simulink model "chap4_3sim"  (Simulink 6.3)
settings: Solver=ode45  StartTime=0.0  StopTime=10  FixedStep=0.001  RelTol=1e-3
libraries: simulink x1
settings Model: LastModifiedBy=Administrator  ExtModeTrigMode=oneshot  ExtModeArmWhenConnect=off  StrictBusMsg=None
settings DataIOCC: LimitDataPoints=off  SignalLoggingName=sigsOut
settings OptimizationCC: BooleanDataType=off
settings DebuggingCC: SolverPrmCheckMsg=none
settings HardwareCC: TargetUnknown=on

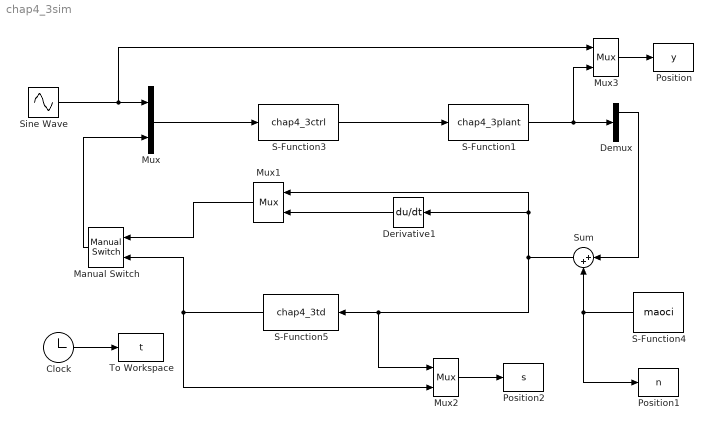
== system chap4_3sim ==
  Clock : Clock
      settings: Decimation=10
  Demux : Demux  Outputs=2
  Derivative1 : Derivative  Orientation=left
  Manual Switch : simulink/Signal Routing/Manual Switch  Orientation=left  sw=0  action=0
  Mux : Mux  Inputs=2
  Mux1 : Mux  Orientation=left  Inputs=2
  Mux2 : Mux  Inputs=2
  Mux3 : Mux  Inputs=2
  Position : ToWorkspace  VariableName=y  SampleTime=-1  SaveFormat=Array
  Position1 : ToWorkspace  VariableName=n  SampleTime=-1  SaveFormat=Array
  Position2 : ToWorkspace  VariableName=s  SampleTime=-1  SaveFormat=Array
  S-Function1 : S-Function  FunctionName=chap4_3plant
  S-Function3 : S-Function  FunctionName=chap4_3ctrl
  S-Function4 : S-Function  Orientation=left  FunctionName=maoci
  S-Function5 : S-Function  Orientation=left  FunctionName=chap4_3td
  Sine Wave : Sin  SampleTime=0
  Sum : Sum  Orientation=left  Inputs=|++  SaturateOnIntegerOverflow=on
  To Workspace : ToWorkspace  VariableName=t  SampleTime=-1  SaveFormat=Array
  wires:
  Sine Wave/1 -> Mux3/1, Mux/1
  Mux3/1 -> Position/1
  S-Function3/1 -> S-Function1/1
  Clock/1 -> To Workspace/1
  S-Function4/1 -> Sum/2, Position1/1
  Sum/1 -> Mux1/1, Derivative1/1, Mux2/1, S-Function5/1
  Mux/1 -> S-Function3/1
  Manual Switch/1 -> Mux/2
  S-Function5/1 -> Manual Switch/2, Mux2/2
  Mux1/1 -> Manual Switch/1
  Derivative1/1 -> Mux1/2
  Mux2/1 -> Position2/1
  S-Function1/1 -> Demux/1, Mux3/2
  Demux/1 -> Sum/1
